simulink model "RealEstadoServoTipo0Obser"  (R2021b)
settings: Solver=VariableStepAuto  StartTime=0.0  StopTime=10.0  RelTol=1e-3
values from neighbouring files (symbols this model uses):
  A = sys.A    [RealEstadoObserServoTipo0.m]
  B = sys.B    [RealEstadoObserServoTipo0.m]
  C = sys.C    [RealEstadoObserServoTipo0.m]    (also in control 2 tf.mat = 0.0033)
  K = Khat(1:m-1)    [RealEstadoObserServoTipo0.m]
  Ke = acker(A',C',[-30 -30 -30])'    [RealEstadoObserServoTipo0.m]
  Ki = -Khat(m)    [RealEstadoObserServoTipo0.m]
settings Model: Creator=mluser  LastModifiedBy=mluser

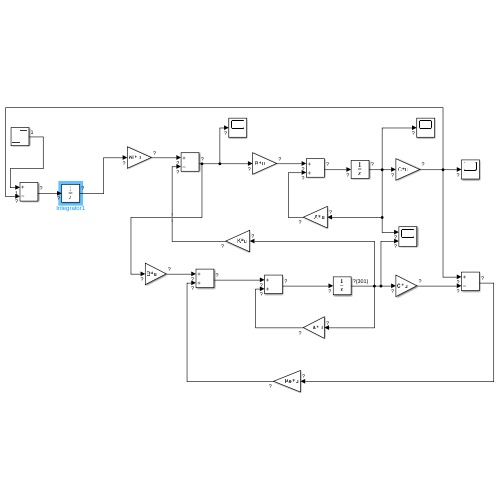
[thumbnail: Simulink's stored preview of the top-level diagram]
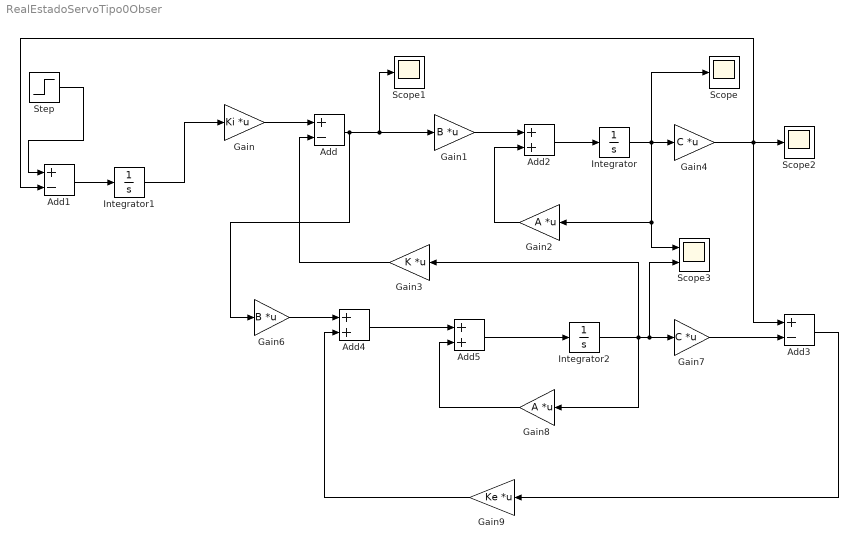
== system RealEstadoServoTipo0Obser ==
  Add : Sum  Inputs=+-
  Add1 : Sum  Inputs=+-
  Add2 : Sum
  Add3 : Sum  Inputs=+-
  Add4 : Sum
  Add5 : Sum
  Gain : Gain  Gain=Ki  Multiplication=Matrix(K*u)
  Gain1 : Gain  Gain=B  Multiplication=Matrix(K*u)
  Gain2 : Gain  Gain=A  Multiplication=Matrix(K*u)
  Gain3 : Gain  Gain=K  Multiplication=Matrix(K*u)
  Gain4 : Gain  Gain=C  Multiplication=Matrix(K*u)
  Gain6 : Gain  Gain=B  Multiplication=Matrix(K*u)
  Gain7 : Gain  Gain=C  Multiplication=Matrix(K*u)
  Gain8 : Gain  Gain=A  Multiplication=Matrix(K*u)
  Gain9 : Gain  Gain=Ke  Multiplication=Matrix(K*u)
  Integrator : Integrator
  Integrator1 : Integrator
  Integrator2 : Integrator
  Scope : Scope
  Scope1 : Scope
  Scope2 : Scope
  Scope3 : Scope  NumInputPorts=2
  Step : Step  Time=0  SampleTime=0
  wires:
  Gain1/1 -> Add2/1
  Integrator1/1 -> Gain/1
  Gain4/1 -> Add1/2, Scope2/1, Add3/1
  Step/1 -> Add1/1
  Integrator/1 -> Scope3/1, Gain2/1, Gain4/1, Scope/1
  Add/1 -> Gain6/1, Scope1/1, Gain1/1
  Gain/1 -> Add/1
  Add2/1 -> Integrator/1
  Gain3/1 -> Add/2
  Gain2/1 -> Add2/2
  Add1/1 -> Integrator1/1
  Integrator2/1 -> Gain3/1, Scope3/2, Gain7/1, Gain8/1
  Gain6/1 -> Add4/1
  Gain8/1 -> Add5/2
  Add4/1 -> Add5/1
  Gain7/1 -> Add3/2
  Add5/1 -> Integrator2/1
  Gain9/1 -> Add4/2
  Add3/1 -> Gain9/1
